simulink model "block_dia_op_strat"  (R2016a)
settings: Solver=VariableStepAuto  StartTime=0.0  StopTime=10.0  RelTol=1e-3
undefined symbols (not defined in the file): chi
settings Model: Creator=sebastian  LastModifiedBy=sebastian

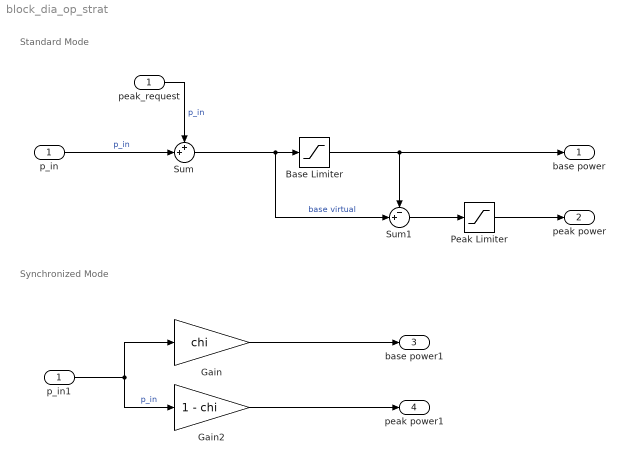
== system block_dia_op_strat ==
  note: Standard Mode
  note: Synchronized Mode
  p_in : Inport
  Base Limiter : Saturate
  Gain : Gain  Gain=chi
  Gain2 : Gain  Gain=1 - chi
  Peak Limiter : Saturate
  Sum : Sum  Inputs=++|
  Sum1 : Sum  Inputs=-+|
  p_in1 : InportShadow
  peak_request : InportShadow
  base power : Outport
  peak power : Outport  Port=2
  base power1 : Outport  Port=3
  peak power1 : Outport  Port=4
  wires:
  p_in/1 -> Sum/2  "p_in"
  peak_request/1 -> Sum/1  "p_in"
  Sum/1 -> Sum1/2, Base Limiter/1  "base virtual"
  Base Limiter/1 -> Sum1/1, base power/1
  Sum1/1 -> Peak Limiter/1
  Peak Limiter/1 -> peak power/1
  Gain/1 -> base power1/1
  Gain2/1 -> peak power1/1
  p_in1/1 -> Gain/1, Gain2/1  "p_in"
